simulink model "mecatronica"  (R2015a)
settings: Solver=ode45  StartTime=0.0  StopTime=2  RelTol=1e-3
values from neighbouring files (symbols this model uses):
  den = conv([1 2],[1 3])    [mecatronica.m]
  num = [1]    [mecatronica.m]
  Ts = 0.02    [mecatronica.m]
undefined symbols (not defined in the file or in its folder): dend, numd
libraries: simulink x2
settings Model: Creator=R_V  LastModifiedBy=R_V

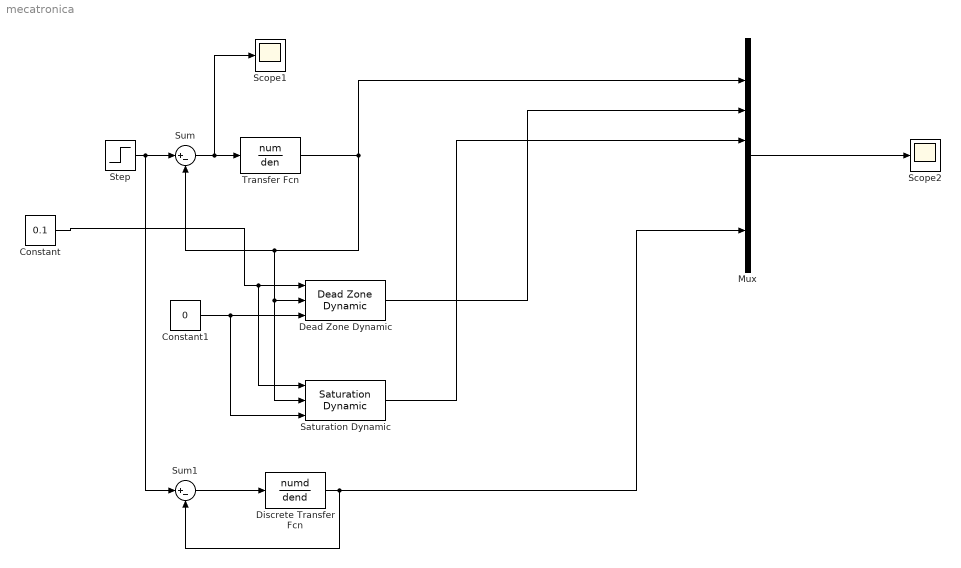
== system mecatronica ==
  Constant : Constant  Value=0.1
  Constant1 : Constant  Value=0
  Dead Zone Dynamic : simulink/Discontinuities/Dead Zone Dynamic
  Discrete Transfer Fcn : DiscreteTransferFcn  Numerator=numd  Denominator=dend  SampleTime=Ts
  Mux : Mux  Inputs=8
  Saturation Dynamic : simulink/Discontinuities/Saturation Dynamic  OutMin=[]  OutMax=[]  OutDataTypeStr=Inherit: Same as second input  OutDataType=fixdt(1, 16)  OutScaling=2^-10  DoSatur=off
  Scope1 : Scope
  Scope2 : Scope
      settings: SaveName=ScopeData2
  Step : Step  Time=0  SampleTime=0
  Sum : Sum  Inputs=|+-
  Sum1 : Sum  Inputs=|+-
  Transfer Fcn : TransferFcn  Numerator=num  Denominator=den
  wires:
  Transfer Fcn/1 -> Mux/2, Dead Zone Dynamic/2, Saturation Dynamic/2, Sum/2
  Constant1/1 -> Saturation Dynamic/3, Dead Zone Dynamic/3
  Constant/1 -> Saturation Dynamic/1, Dead Zone Dynamic/1
  Sum/1 -> Scope1/1, Transfer Fcn/1
  Mux/1 -> Scope2/1
  Step/1 -> Sum1/1, Sum/1
  Sum1/1 -> Discrete Transfer Fcn/1
  Discrete Transfer Fcn/1 -> Mux/7, Sum1/2
  Dead Zone Dynamic/1 -> Mux/3
  Saturation Dynamic/1 -> Mux/4
